simulink model "vozidla3_komplet"  (R2021a)
settings: Solver=VariableStepAuto  StartTime=0.0  StopTime=80  RelTol=1e-9
values from neighbouring files (symbols this model uses):
  A = A(1:(numOfStates),1:(numOfStates))    [systemGen.m]
  B = zeros(numOfStates,N)    [systemGen.m]
  C = {'c','m','r','b','g',[0.4660 0.6740 0.1880],'y',[0.6350 0.0780 0.1840],[0 0.4470 0.7410],[0.9290 0.6940 0.1250]}    [hl_script_rozsireniBP.m]    (also in systemGen.m = eye(numOfStates))
  conds = zeros(1,numOfStates)    [hl_script_rozsireniBP.m]
  Cw = Cw1    [hl_script_rozsireniBP.m]
  Cy = zeros(N,numOfStates)    [systemGen.m]
  D = zeros(numOfStates,N)    [systemGen.m]
  eigenvals = [p q r]    [hl_script_rozsireniBP.m]
  inputDist = 1    [hl_script_rozsireniBP.m]
  K = symFgen(N,numOfStates,eigenvals,structure,A,B)    [hl_script_rozsireniBP.m]
  setpoints = zeros(numOfStates,1)    [hl_script_rozsireniBP.m]
  structure = 5    [hl_script_rozsireniBP.m]
libraries: simulink x1
settings Model: PacingRate=0.500000  Creator=radek  LastModifiedBy=radek

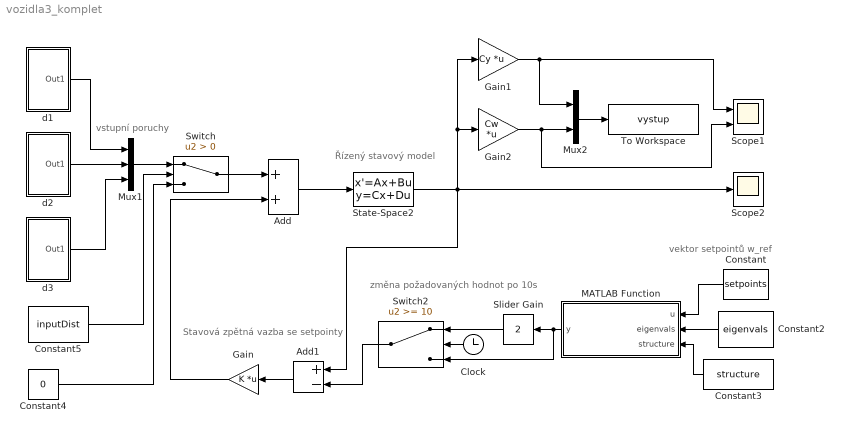
== system vozidla3_komplet ==
  note: změna požadovaných hodnot po 10s
  note: Stavová zpětná vazba se setpointy
  note: vektor setpointů w_ref
  note: vstupní poruchy
  note: Řízený stavový model
  Add : Sum
  Add1 : Sum  Inputs=+-
  Clock : Clock
  Constant : Constant  Value=setpoints
  Constant2 : Constant  Value=eigenvals
  Constant3 : Constant  Value=structure
  Constant4 : Constant  Value=0
  Constant5 : Constant  Value=inputDist
  Gain : Gain  Gain=K  Multiplication=Matrix(K*u)
  Gain1 : Gain  Gain=Cy  Multiplication=Matrix(K*u)
  Gain2 : Gain  Gain=Cw  Multiplication=Matrix(K*u)
  MATLAB Function : MATLAB Function  TreatAsAtomicUnit=on
  Mux1 : Mux  Inputs=3
  Mux2 : Mux  Inputs=2
  Scope1 : Scope  NumInputPorts=2
  Scope2 : Scope
  Slider Gain : simulink/Math Operations/Slider Gain  gain=2  low=0  high=4
  State-Space2 : StateSpace  A=A  B=B  C=C  D=D  InitialCondition=conds  ParameterTunability=Optimized
  Switch : Switch  Criteria=u2 > Threshold
  Switch2 : Switch  Threshold=10
  To Workspace : ToWorkspace  VariableName=vystup  SaveFormat=Structure  SampleTime=-1
  d1 : Subsystem
  d2 : Subsystem
  d3 : Subsystem
  wires:
  d1/1(Out1) -> Mux1/1
  d2/1(Out1) -> Mux1/2
  d3/1(Out1) -> Mux1/3
  Add/1 -> State-Space2/1
  Gain/1 -> Add/2
  State-Space2/1 -> Add1/1, Scope2/1, Gain1/1, Gain2/1
  Gain1/1 -> Scope1/1, Mux2/1
  Gain2/1 -> Scope1/2, Mux2/2
  Add1/1 -> Gain/1
  Constant/1 -> MATLAB Function/1(u)
  Constant2/1 -> MATLAB Function/2(eigenvals)
  Constant3/1 -> MATLAB Function/3(structure)
  Constant5/1 -> Switch/2
  Switch/1 -> Add/1
  Mux1/1 -> Switch/1
  Constant4/1 -> Switch/3
  Switch2/1 -> Add1/2
  Mux2/1 -> To Workspace/1
  MATLAB Function/1(y) -> Switch2/3, Slider Gain/1
  Slider Gain/1 -> Switch2/1
  Clock/1 -> Switch2/2

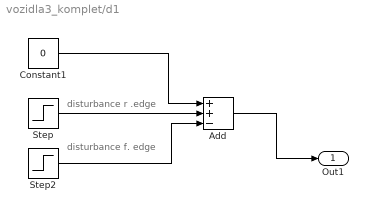
== system vozidla3_komplet/d1 ==
  note: disturbance f. edge
  note: disturbance r .edge
  Add : Sum  Inputs=++-
  Constant1 : Constant  Value=0
  Step : Step  Time=5  After=2  SampleTime=0
  Step2 : Step  Time=6  After=2  SampleTime=0
  Out1 : Outport
  wires:
  Constant1/1 -> Add/1
  Add/1 -> Out1/1
  Step/1 -> Add/2
  Step2/1 -> Add/3

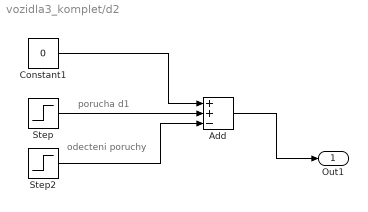
== system vozidla3_komplet/d2 ==
  note: odecteni poruchy
  note: porucha d1
  Add : Sum  Inputs=++-
  Constant1 : Constant  Value=0
  Step : Step  Time=25  After=2  SampleTime=0
  Step2 : Step  Time=26  After=2  SampleTime=0
  Out1 : Outport
  wires:
  Constant1/1 -> Add/1
  Step2/1 -> Add/3
  Add/1 -> Out1/1
  Step/1 -> Add/2

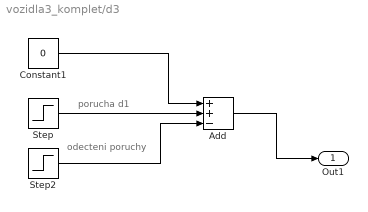
== system vozidla3_komplet/d3 ==
  note: odecteni poruchy
  note: porucha d1
  Add : Sum  Inputs=++-
  Constant1 : Constant  Value=0
  Step : Step  Time=45  After=2  SampleTime=0
  Step2 : Step  Time=46  After=2  SampleTime=0
  Out1 : Outport
  wires:
  Constant1/1 -> Add/1
  Step2/1 -> Add/3
  Add/1 -> Out1/1
  Step/1 -> Add/2

== matlab function vozidla3_komplet/MATLAB Function ==
  data: u input; y output; eigenvals input; structure input
function y = Pgain(u,eigenvals,structure)
lambda = eigenvals(1);
nu = eigenvals(2);
if structure == 1
    temp = lambda/(lambda-1);
elseif structure == 2  
    temp = nu/(nu-1);
elseif structure == 3
    if lambda == nu
        temp = (lambda+nu)/(lambda+nu-2);
    else
        temp = lambda/(lambda-1);
    end
elseif structure == 5
    % lqr
    if eigenvals(3) == 1
        temp = (eigenvals(1)+1)/(eigenvals(1));
    else
        temp = (eigenvals(1)+1)/eigenvals(3);
% temp = 1;
    end
else
    temp = 1;
end
u(1:2:length(u)) = u(1:2:length(u))*temp;
y = u;
